simulink model "InitialSystem_9_Bus"  (R2020a)
settings: Solver=FixedStepAuto  StartTime=0.0  StopTime=Tend  MaxStep=5.0E-5  RelTol=1e-3
values from neighbouring files (symbols this model uses):
  B_s46 = b_s46*Cb    (= 9.5071761847e-07)    [Data_CaseStudyI.m]    (also in Data_CaseStudyII.m; Data_InitialSystem.m)
  B_s54 = b_s54*Cb    (= 1.05902722057e-06)    [Data_CaseStudyI.m]    (also in Data_CaseStudyII.m; Data_InitialSystem.m)
  B_s69 = b_s69*Cb    (= 2.15415764185e-06)    [Data_CaseStudyI.m]    (also in Data_CaseStudyII.m; Data_InitialSystem.m)
  B_s75 = b_s75*Cb    (= 1.84126323577e-06)    [Data_CaseStudyI.m]    (also in Data_CaseStudyII.m; Data_InitialSystem.m)
  B_s87 = b_s87*Cb    (= 8.96562817417e-07)    [Data_CaseStudyI.m]    (also in Data_CaseStudyII.m; Data_InitialSystem.m)
  B_s98 = b_s98*Cb    (= 1.25759482443e-06)    [Data_CaseStudyI.m]    (also in Data_CaseStudyII.m; Data_InitialSystem.m)
  fb = 50    [Data_CaseStudyI.m]    (also in Data_CaseStudyII.m; Data_InitialSystem.m)
  HGov_dyn = HGov_delay*H_tr_droop    [Data_CaseStudyI.m]    (also in Data_CaseStudyII.m; Data_InitialSystem.m)
  HTurb_tot = H_water_way    [Data_CaseStudyI.m]    (also in Data_CaseStudyII.m; Data_InitialSystem.m)
  l1_MVHV1 = 0    [Data_CaseStudyI.m]    (also in Data_CaseStudyII.m; Data_InitialSystem.m)
  l1_MVHV2 = 0    [Data_CaseStudyI.m]    (also in Data_CaseStudyII.m; Data_InitialSystem.m)
  l1_MVHV3 = 0    [Data_CaseStudyI.m]    (also in Data_CaseStudyII.m; Data_InitialSystem.m)
  l2_MVHV1 = l_s14    (= 0.0576)    [Data_CaseStudyI.m]    (also in Data_CaseStudyII.m; Data_InitialSystem.m)
  l2_MVHV2 = l_s72    (= 0.0625)    [Data_CaseStudyI.m]    (also in Data_CaseStudyII.m; Data_InitialSystem.m)
  l2_MVHV3 = l_s39    (= 0.0586)    [Data_CaseStudyI.m]    (also in Data_CaseStudyII.m; Data_InitialSystem.m)
  L_s46 = l_s46*Lb    (= 0.154915055408)    [Data_CaseStudyI.m]    (also in Data_CaseStudyII.m; Data_InitialSystem.m)
  L_s54 = l_s54*Lb    (= 0.143128040323)    [Data_CaseStudyI.m]    (also in Data_CaseStudyII.m; Data_InitialSystem.m)
  L_s69 = l_s69*Lb    (= 0.286256080645)    [Data_CaseStudyI.m]    (also in Data_CaseStudyII.m; Data_InitialSystem.m)
  L_s75 = l_s75*Lb    (= 0.271101346964)    [Data_CaseStudyI.m]    (also in Data_CaseStudyII.m; Data_InitialSystem.m)
  L_s87 = l_s87*Lb    (= 0.12123786945)    [Data_CaseStudyI.m]    (also in Data_CaseStudyII.m; Data_InitialSystem.m)
  L_s98 = l_s98*Lb    (= 0.16973301723)    [Data_CaseStudyI.m]    (also in Data_CaseStudyII.m; Data_InitialSystem.m)
  P_L = pL*Sb    (= 300000000)    [Data_CaseStudyI.m]    (also in Data_CaseStudyII.m; Data_InitialSystem.m)
  p_set_bus1 = P_set_bus1/SbSG1    (= 0.731707317073)    [Data_CaseStudyI.m]    (also in Data_CaseStudyII.m; Data_InitialSystem.m)
  p_set_bus2 = P_set_bus2/SbSG2    (= 0.756707317073)    [Data_CaseStudyI.m]    (also in Data_CaseStudyII.m; Data_InitialSystem.m)
  p_set_bus3 = P_set_bus3/SbSG3    (= 0.731707317073)    [Data_CaseStudyI.m]    (also in Data_CaseStudyII.m; Data_InitialSystem.m)
  Q_L = qL*Sb    (= 82500000)    [Data_CaseStudyI.m]    (also in Data_CaseStudyII.m; Data_InitialSystem.m)
  r1_MVHV1 = 1e-6    (= 1e-06)    [Data_CaseStudyI.m]    (also in Data_CaseStudyII.m; Data_InitialSystem.m)
  r1_MVHV2 = 1e-6    (= 1e-06)    [Data_CaseStudyI.m]    (also in Data_CaseStudyII.m; Data_InitialSystem.m)
  r1_MVHV3 = 1e-6    (= 1e-06)    [Data_CaseStudyI.m]    (also in Data_CaseStudyII.m; Data_InitialSystem.m)
  r2_MVHV1 = 1e-6    (= 1e-06)    [Data_CaseStudyI.m]    (also in Data_CaseStudyII.m; Data_InitialSystem.m)
  r2_MVHV2 = 1e-6    (= 1e-06)    [Data_CaseStudyI.m]    (also in Data_CaseStudyII.m; Data_InitialSystem.m)
  r2_MVHV3 = 1e-6    (= 1e-06)    [Data_CaseStudyI.m]    (also in Data_CaseStudyII.m; Data_InitialSystem.m)
  R_s46 = r_s46*Zb    (= 8.993)    [Data_CaseStudyI.m]    (also in Data_CaseStudyII.m; Data_InitialSystem.m)
  R_s54 = r_s54*Zb    (= 5.29)    [Data_CaseStudyI.m]    (also in Data_CaseStudyII.m; Data_InitialSystem.m)
  R_s69 = r_s69*Zb    (= 20.631)    [Data_CaseStudyI.m]    (also in Data_CaseStudyII.m; Data_InitialSystem.m)
  R_s75 = r_s75*Zb    (= 16.928)    [Data_CaseStudyI.m]    (also in Data_CaseStudyII.m; Data_InitialSystem.m)
  R_s87 = r_s87*Zb    (= 4.4965)    [Data_CaseStudyI.m]    (also in Data_CaseStudyII.m; Data_InitialSystem.m)
  R_s98 = r_s98*Zb    (= 6.2951)    [Data_CaseStudyI.m]    (also in Data_CaseStudyII.m; Data_InitialSystem.m)
  Rg = 0.03    [Data_CaseStudyI.m]    (also in Data_CaseStudyII.m; Data_InitialSystem.m)
  Sb = 100*10^6    (= 100000000)    [Data_CaseStudyI.m]    (also in Data_CaseStudyII.m; Data_InitialSystem.m)
  SbSG1 = r_b1*100*10^6    (= 250000000)    [Data_CaseStudyI.m]    (also in Data_CaseStudyII.m; Data_InitialSystem.m)
  SbSG2 = r_b2*100*10^6    (= 96000000)    [Data_CaseStudyI.m]    (also in Data_CaseStudyII.m; Data_InitialSystem.m)
  SbSG3 = r_b3*100*10^6    (= 64000000)    [Data_CaseStudyI.m]    (also in Data_CaseStudyII.m; Data_InitialSystem.m)
  SGov_dyn = tf([1],[Tg 1])    [Data_CaseStudyI.m]    (also in Data_CaseStudyII.m; Data_InitialSystem.m)
  St_MVHV1 = Sb    (= 100000000)    [Data_CaseStudyI.m]    (also in Data_CaseStudyII.m; Data_InitialSystem.m)
  St_MVHV2 = Sb    (= 100000000)    [Data_CaseStudyI.m]    (also in Data_CaseStudyII.m; Data_InitialSystem.m)
  St_MVHV3 = Sb    (= 100000000)    [Data_CaseStudyI.m]    (also in Data_CaseStudyII.m; Data_InitialSystem.m)
  STurb_reheat = STurb_ch*STurb_rh    [Data_CaseStudyI.m]    (also in Data_CaseStudyII.m; Data_InitialSystem.m)
  T_load_b6 = 1010    [Data_CaseStudyI.m]    (also in Data_InitialSystem.m)
  T_s_power = 1e-4    (= 0.0001)    [Data_CaseStudyI.m]    (also in Data_CaseStudyII.m; Data_InitialSystem.m)
  VbHV = 230*10^3    (= 230000)    [Data_CaseStudyI.m]    (also in Data_CaseStudyII.m; Data_InitialSystem.m)
  VbMV1 = 16.5*10^3    (= 16500)    [Data_CaseStudyI.m]    (also in Data_CaseStudyII.m; Data_InitialSystem.m)
  VbMV2 = 18.0*10^3    (= 18000)    [Data_CaseStudyI.m]    (also in Data_CaseStudyII.m; Data_InitialSystem.m)
  VbMV3 = 13.8*10^3    (= 13800)    [Data_CaseStudyI.m]    (also in Data_CaseStudyII.m; Data_InitialSystem.m)
undefined symbols (not defined in the file or in its folder): A, B, C, Continuous, Dd, Efd0, gcbh, Ka, Kf, p2set, SbSM2, sps_rtmsupport, spsST1AModel, Ta, Tb, Tb1, Tc, Tc1, Tf, VA0, VAmax, VAmin, VImax, VImin, VRmax, VRmin
libraries: powerlib x55, cstblocks x6, sps_avr x2, simulink_extras x1, simulink x1
(part 2 of 2)

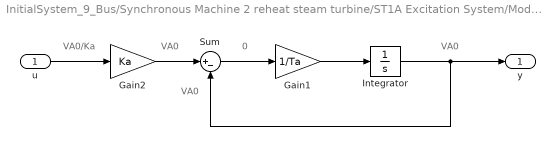
== system InitialSystem_9_Bus/Synchronous Machine 2 reheat steam turbine/ST1A Excitation System/Model/Vaminmax ==
  note: VA0/Ka
  note: VA0
  note: VA0
  note: 0
  note: VA0
  u : Inport
  Gain1 : Gain  Gain=1/Ta  SaturateOnIntegerOverflow=on  OutDataTypeStr=Inherit: Same as input  ParamDataTypeStr=Inherit: Same as input
  Gain2 : Gain  Gain=Ka  SaturateOnIntegerOverflow=on  OutDataTypeStr=Inherit: Same as input  ParamDataTypeStr=Inherit: Same as input
  Integrator : Integrator  InitialCondition=VA0  LimitOutput=on  UpperSaturationLimit=VAmax  LowerSaturationLimit=VAmin
  Sum : Sum  Inputs=|+-  InputSameDT=on  SaturateOnIntegerOverflow=on  OutDataTypeStr=Inherit: Same as first input
  y : Outport
  wires:
  u/1 -> Gain2/1
  Sum/1 -> Gain1/1
  Integrator/1 -> y/1, Sum/2
  Gain2/1 -> Sum/1
  Gain1/1 -> Integrator/1
